simulink model "UR5_SDH_IK"  (R2023b)
settings: Solver=VariableStepAuto  StartTime=0.0  StopTime=10.0  RelTol=1e-3
values from neighbouring files (symbols this model uses):
  R = [1 0 0 ... (first row only)    [Main.m]
  T = transl(P(i,:)) * rpy2tr(0, 0, pi, 'xyz')    [Gluon6L3.m]    (also in Main.m = [     -0.09743  -0.8140    0.5726   -0.1557; UR5_Heart.m = transl(P(i,: )) * rpy2tr(0, pi/4, pi, 'xyz'); drawCircle.m = [R_goal,      P(i,:)')
undefined symbols (not defined in the file or in its folder): smiData, X, Y, Z
libraries: sm_lib x136, fl_lib x25, nesl_utility x14, robotcorelib x2
(part 3 of 3)

== system UR5_SDH_IK/Robot/robot/J6_1_RIGID/x33103_1_RIGID ==
  ReferenceFrame : sm_lib/Frames and Transforms/Reference Frame
  Solid : sm_lib/Body Elements/File Solid  ExtGeomFileName=33103_Default_sldprt.STEP  UnitType=FromFile  ExtGeomFileUnits=m  StepReaderType=HEX  ExportConvexHullGeometry=off  InertiaType=Custom  Mass=smiData.Solid(15).mass  MassUnits=kg  CenterOfMass=smiData.Solid(15).CoM  CenterOfMassUnits=cm  MomentsOfInertia=smiData.Solid(15).MoI  MomentsOfInertiaUnits=kg*cm^2  ProductsOfInertia=smiData.Solid(15).PoI  ProductsOfInertiaUnits=kg*cm^2  BasedOnType=DensityFromFile  Density=1000  DensityUnits=kg/m^3  DoExposeReferenceFrame=on  SerializedFrames=<Frames/>  GraphicType=FromGeometry  MarkerShape=Sphere  MarkerSize=10  GraphicVisPropType=SimpleVisualProperties  GraphicDiffuseColor=smiData.Solid(15).color  GraphicSpecularColor=[0.5 0.5 0.5 1.0]  GraphicAmbientColor=[0.15 0.15 0.15 1.0]  GraphicEmissiveColor=[0.0 0.0 0.0 1.0]  GraphicShininess=75  GraphicOpacity=smiData.Solid(15).opacity
  F : PMIOPort  Side=Left
  connections:
  Solid/RConn1 -- ReferenceFrame/RConn1 -- F/RConn1

== system UR5_SDH_IK/Robot/robot/J6_1_RIGID/x33116_1_RIGID ==
  ReferenceFrame : sm_lib/Frames and Transforms/Reference Frame
  Solid : sm_lib/Body Elements/File Solid  ExtGeomFileName=33116_Default_sldprt.STEP  UnitType=FromFile  ExtGeomFileUnits=m  StepReaderType=HEX  ExportConvexHullGeometry=off  InertiaType=Custom  Mass=smiData.Solid(14).mass  MassUnits=kg  CenterOfMass=smiData.Solid(14).CoM  CenterOfMassUnits=cm  MomentsOfInertia=smiData.Solid(14).MoI  MomentsOfInertiaUnits=kg*cm^2  ProductsOfInertia=smiData.Solid(14).PoI  ProductsOfInertiaUnits=kg*cm^2  BasedOnType=DensityFromFile  Density=1000  DensityUnits=kg/m^3  DoExposeReferenceFrame=on  SerializedFrames=<Frames/>  GraphicType=FromGeometry  MarkerShape=Sphere  MarkerSize=10  GraphicVisPropType=SimpleVisualProperties  GraphicDiffuseColor=smiData.Solid(14).color  GraphicSpecularColor=[0.5 0.5 0.5 1.0]  GraphicAmbientColor=[0.15 0.15 0.15 1.0]  GraphicEmissiveColor=[0.0 0.0 0.0 1.0]  GraphicShininess=75  GraphicOpacity=smiData.Solid(14).opacity
  F : PMIOPort  Side=Left
  connections:
  Solid/RConn1 -- ReferenceFrame/RConn1 -- F/RConn1

== matlab function UR5_SDH_IK/FK/MATLAB Function ==
  data: theta input; T output
function T = zhengyundongxue(theta)
    %已知关节角求变换矩阵
    a=[0,-0.42500,-0.39225,0,0,0];
    d=[0.089159,0,0,0.10915,0.09465,0.08230];
    alpha=[pi/2,0,0,pi/2,-pi/2,0];
 
    
    T01=T_para(theta(1),d(1),a(1),alpha(1));
    T12=T_para(theta(2),d(2),a(2),alpha(2));
    T23=T_para(theta(3),d(3),a(3),alpha(3));
    T34=T_para(theta(4),d(4),a(4),alpha(4));
    T45=T_para(theta(5),d(5),a(5),alpha(5));
    T56=T_para(theta(6),d(6),a(6),alpha(6));
    
    T=T01*T12*T23*T34*T45*T56;
    
end
 
function T = T_para(theta,d,a,alpha)
    T=[ccc(theta),-sss(theta)*ccc(alpha),sss(theta)*sss(alpha),a*ccc(theta);
        sss(theta),ccc(theta)*ccc(alpha),-ccc(theta)*sss(alpha),a*sss(theta);
        0,sss(alpha),ccc(alpha),d;
        0,0,0,1];
end
 
function sss=sss(a)
%     sss=sin(a/180*pi);
    sss=sin(a);
end
 
function ccc=ccc(a)
%     ccc=cos(a/180*pi);
     ccc=cos(a);
end

== matlab function UR5_SDH_IK/MATLAB Function ==
  data: p input; T output; R input
function T = BuildT(p, R)
% BuildT  根据固定旋转矩阵 R 和输入位置 p 构建齐次变换矩阵 T
% 输入:
%   p[3x1] - 末端位置向量 [x; y; z]
% 输出:
%   T[4x4] - 齐次变换矩阵

% 固定旋转矩阵 R
% R = [0, 0, 1;
%      0, -1, 0;
%      1, 0, 0];

% 构建齐次矩阵
T = [R, p(:);     % p(:) 确保为列向量
     0 0 0 1];

end

== matlab function UR5_SDH_IK/MATLAB Function1 ==
  data: T input; joint_angles output
function joint_angles = ur5_inverse_kinematics(T)
%#codegen
%UR5_INVERSE_KINEMATICS UR5机械臂逆运动学解析解（Simulink MATLAB Function兼容）
%
%   输入:  
%       T           - 4x4 齐次变换矩阵，表示末端执行器位姿
%
%   输出:
%       joint_angles - 8x6 矩阵，每行为一组可能的关节角解 [θ1,θ2,θ3,θ4,θ5,θ6] (rad)
%
%   说明:
%       基于UR5标准DH参数:  alpha = [pi/2, 0, 0, pi/2, -pi/2, 0]
%       共有8组解，对应不同的机械臂配置（肩部左/右、肘部上/下、腕部翻转）

    %% ================== UR5 DH参数定义 ==================
    % 连杆长度 (单位: m)
    LINK_A2 = -0.42500;     % 连杆2长度 (上臂)
    LINK_A3 = -0.39225;     % 连杆3长度 (前臂)
    
    % 连杆偏移 (单位: m)
    OFFSET_D1 = 0.089159;   % 基座到关节1的偏移
    OFFSET_D4 = 0.10915;    % 关节3到关节4的偏移
    OFFSET_D5 = 0.09465;    % 关节4到关节5的偏移
    OFFSET_D6 = 0.08230;    % 关节5到末端的偏移

    %% ================== 提取变换矩阵元素 ==================
    % 旋转矩阵 R = [n, o, a]
    % n: 法向量(normal), o: 方向向量(orientation), a: 接近向量(approach)
    nx = T(1,1);  ny = T(2,1);  nz = T(3,1);    % 法向量
    ox = T(1,2);  oy = T(2,2);  oz = T(3,2);    % 方向向量
    ax = T(1,3);  ay = T(2,3);  az = T(3,3);    % 接近向量
    
    % 位置向量 p
    px = T(1,4);  py = T(2,4);  pz = T(3,4);

    %% ================== 初始化所有变量 ==================
    % Simulink代码生成要求：所有数组必须先完整初始化
    joint_angles = zeros(8, 6);
    theta1_sol = zeros(1, 2);
    theta5_sol = zeros(2, 2);
    theta6_sol = zeros(2, 2);
    P14_x = zeros(2, 2);
    P14_z = zeros(2, 2);
    cos_theta3 = zeros(2, 2);
    theta3_sol_pos = zeros(2, 2);
    theta3_sol_neg = zeros(2, 2);
    theta2_sol = zeros(2, 2, 2);

    %% ================== 求解关节角1 (θ1) ==================
    % 计算腕心位置在XY平面的投影
    wrist_center_y = OFFSET_D6 * ay - py;
    wrist_center_x = OFFSET_D6 * ax - px;
    
    % 计算辅助角度和距离
    psi = atan2(wrist_center_y, wrist_center_x);
    
    % 防止数值误差导致负数开方
    dist_squared = wrist_center_x^2 + wrist_center_y^2 - OFFSET_D4^2;
    if dist_squared < 0
        dist_squared = 0;
    end
    radial_dist = sqrt(dist_squared);
    
    % θ1的两个解 (左肩/右肩配置)
    theta1_sol(1) = psi - atan2(OFFSET_D4,  radial_dist);
    theta1_sol(2) = psi - atan2(OFFSET_D4, -radial_dist);

    %% ================== 求解关节角5 (θ5) ==================
    % 对每个θ1计算θ5
    cos_theta5_1 = ax * sin(theta1_sol(1)) - ay * cos(theta1_sol(1));
    cos_theta5_2 = ax * sin(theta1_sol(2)) - ay * cos(theta1_sol(2));
    
    % 限制cos值在[-1, 1]范围内
    if cos_theta5_1 > 1
        cos_theta5_1 = 1;
    elseif cos_theta5_1 < -1
        cos_theta5_1 = -1;
    end
    
    if cos_theta5_2 > 1
        cos_theta5_2 = 1;
    elseif cos_theta5_2 < -1
        cos_theta5_2 = -1;
    end
    
    % θ5的四个解 (腕部正/反配置)
    % theta5_sol(i,j): i=1,2对应θ1的两个解, j=1,2对应θ5的正负解
    theta5_sol(1,1) =  acos(cos_theta5_1);    % θ1解1, θ5正
    theta5_sol(1,2) = -acos(cos_theta5_1);    % θ1解1, θ5负
    theta5_sol(2,1) =  acos(cos_theta5_2);    % θ1解2, θ5正
    theta5_sol(2,2) = -acos(cos_theta5_2);    % θ1解2, θ5负

    %% ================== 求解关节角6 (θ6) ==================
    % 计算中间变量
    sin_theta6_base1 = nx * sin(theta1_sol(1)) - ny * cos(theta1_sol(1));
    cos_theta6_base1 = ox * sin(theta1_sol(1)) - oy * cos(theta1_sol(1));
    sin_theta6_base2 = nx * sin(theta1_sol(2)) - ny * cos(theta1_sol(2));
    cos_theta6_base2 = ox * sin(theta1_sol(2)) - oy * cos(theta1_sol(2));
    
    % θ6的四个解
    theta6_sol(1,1) = atan2(sin_theta6_base1, cos_theta6_base1) - atan2(sin(theta5_sol(1,1)), 0);
    theta6_sol(1,2) = atan2(sin_theta6_base1, cos_theta6_base1) - atan2(sin(theta5_sol(1,2)), 0);
    theta6_sol(2,1) = atan2(sin_theta6_base2, cos_theta6_base2) - atan2(sin(theta5_sol(2,1)), 0);
    theta6_sol(2,2) = atan2(sin_theta6_base2, cos_theta6_base2) - atan2(sin(theta5_sol(2,2)), 0);

    %% ================== 求解关节角3 (θ3) ==================
    % 计算腕部在关节1坐标系下的位置投影
    for i = 1:2      % 遍历θ1的两个解
        for j = 1:2  % 遍历θ5/θ6的两个解
            c1 = cos(theta1_sol(i));
            s1 = sin(theta1_sol(i));
            c6 = cos(theta6_sol(i,j));
            s6 = sin(theta6_sol(i,j));
            
            % 腕部位置x分量
            P14_x(i,j) = OFFSET_D5 * (s6 * (nx*c1 + ny*s1) + c6 * (ox*c1 + oy*s1)) ... 
                       - OFFSET_D6 * (ax*c1 + ay*s1) + px*c1 + py*s1;
            
            % 腕部位置z分量
            P14_z(i,j) = pz - OFFSET_D1 - az*OFFSET_D6 + OFFSET_D5 * (oz*c6 + nz*s6);
        end
    end
    
    % 使用余弦定理求解θ3
    for i = 1:2
        for j = 1:2
            numerator = P14_x(i,j)^2 + P14_z(i,j)^2 - LINK_A2^2 - LINK_A3^2;
            denominator = 2 * LINK_A2 * LINK_A3;
            cos_theta3(i,j) = numerator / denominator;
            
            % 限制cos值范围
            if cos_theta3(i,j) > 1
                cos_theta3(i,j) = 1;
            elseif cos_theta3(i,j) < -1
                cos_theta3(i,j) = -1;
            end
            
            theta3_sol_pos(i,j) =  acos(cos_theta3(i,j));
            theta3_sol_neg(i,j) = -acos(cos_theta3(i,j));
        end
    end

    %% ================== 求解关节角2 (θ2) ==================
    for i = 1:2
        for j = 1:2
            % θ3为正解时的θ2
            theta2_sol(i,j,1) = calc_theta2_inline(P14_x(i,j), P14_z(i,j), ...
                                                   theta3_sol_pos(i,j), LINK_A2, LINK_A3);
            % θ3为负解时的θ2
            theta2_sol(i,j,2) = calc_theta2_inline(P14_x(i,j), P14_z(i,j), ...
                                                   theta3_sol_neg(i,j), LINK_A2, LINK_A3);
        end
    end

    %% ================== 组装8组解 ==================
    solution_idx = 1;
    for i = 1:2          % θ1索引
        for j = 1:2      % θ5索引
            for k = 1:2  % θ3正负索引
                % 选择对应的θ3
                if k == 1
                    theta3_val = theta3_sol_pos(i,j);
                else
                    theta3_val = theta3_sol_neg(i,j);
                end
                
                % 赋值 θ1, θ2, θ3
                joint_angles(solution_idx, 1) = theta1_sol(i);
                joint_angles(solution_idx, 2) = theta2_sol(i,j,k);
                joint_angles(solution_idx, 3) = theta3_val;
                
                % 赋值 θ5, θ6
                joint_angles(solution_idx, 5) = theta5_sol(i,j);
                joint_angles(solution_idx, 6) = theta6_sol(i,j);
                
                solution_idx = solution_idx + 1;
            end
        end
    end

    %% ================== 求解关节角4 (θ4) ==================
    for sol = 1:8
        t1 = joint_angles(sol, 1);
        t2 = joint_angles(sol, 2);
        t3 = joint_angles(sol, 3);
        t6 = joint_angles(sol, 6);
        
        c1 = cos(t1);
        s1 = sin(t1);
        c6 = cos(t6);
        s6 = sin(t6);
        
        % 计算θ4的sin和cos分量
        sin_theta234 = -s6 * (nx*c1 + ny*s1) - c6 * (ox*c1 + oy*s1);
        cos_theta234 = oz*c6 + nz*s6;
        
        theta234 = atan2(sin_theta234, cos_theta234);
        joint_angles(sol, 4) = theta234 - t2 - t3;
    end

    %% ================== 角度归一化 ==================
    for sol = 1:8
        for jnt = 1:6
            ang = joint_angles(sol, jnt);
            while ang > pi
                ang = ang - 2*pi;
            end
            while ang < -pi
                ang = ang + 2*pi;
            end
            joint_angles(sol, jnt) = ang;
        end
    end

end

%% ================== 内联函数:  计算θ2 ==================
function theta2 = calc_theta2_inline(P14_x, P14_z, theta3, A2, A3)
%CALC_THETA2_INLINE 根据几何关系计算关节角2

    c3 = cos(theta3);
    s3 = sin(theta3);
    
    % 分母
    denom = A2^2 + A3^2 + 2*A2*A3*c3;
    
    % 防止除零
    if abs(denom) < 1e-10
        denom = 1e-10;
    end
    
    % 计算sin(θ2)和cos(θ2)
    sin_theta2 = ((A3*c3 + A2) * P14_z - A3*s3 * P14_x) / denom;
    
    % 防止除零
    denom2 = A3*c3 + A2;
    if abs(denom2) < 1e-10
        denom2 = 1e-10;
    end
    cos_theta2 = (P14_x + A3*s3 * sin_theta2) / denom2;
    
    theta2 = atan2(sin_theta2, cos_theta2);
end

== matlab function UR5_SDH_IK/MATLAB Function2 ==
  data: all_solutions input; optimal_joint output; current_joint input
function optimal_joint = ur5_select_optimal_simple(all_solutions, current_joint)
%#codegen
%UR5_SELECT_OPTIMAL_SIMPLE 从8组逆解中选择最优解（简化版）
%
%   输入:
%       all_solutions - 8x6 矩阵，8组可能的关节角解 (rad)
%       current_joint - 1x6 向量，当前关节角度 (rad)
%
%   输出:
%       optimal_joint - 1x6 向量，最优的关节角解 (rad)
%
%   选择准则:  选择与当前关节角度变化最小的有效解

    %% ================== 初始化 ==================
    NUM_SOLUTIONS = 8;
    NUM_JOINTS = 6;
    
    optimal_joint = zeros(1, NUM_JOINTS);
    min_distance = 1e10;
    best_idx = 0;

    %% ================== 遍历所有解 ==================
    for sol_idx = 1:NUM_SOLUTIONS
        
        % 检查是否为有效解（无NaN/Inf）
        is_valid = true;
        for j = 1:NUM_JOINTS
            if isnan(all_solutions(sol_idx, j)) || isinf(all_solutions(sol_idx, j))
                is_valid = false;
            end
        end
        
        if ~is_valid
            continue;
        end
        
        % 计算与当前关节角度的距离
        distance = 0;
        for j = 1:NUM_JOINTS
            % 角度差归一化
            diff = all_solutions(sol_idx, j) - current_joint(j);
            
            while diff > pi
                diff = diff - 2*pi;
            end
            while diff < -pi
                diff = diff + 2*pi;
            end
            
            distance = distance + diff^2;
        end
        distance = sqrt(distance);
        
        % 更新最优解
        if distance < min_distance
            min_distance = distance;
            best_idx = sol_idx;
        end
    end

    %% ================== 输出结果 ==================
    if best_idx > 0
        for j = 1:NUM_JOINTS
            ang = all_solutions(best_idx, j);
            while ang > pi
                ang = ang - 2*pi;
            end
            while ang < -pi
                ang = ang + 2*pi;
            end
            optimal_joint(j) = ang;
        end
    else
        % 无有效解，返回当前角度
        for j = 1:NUM_JOINTS
            optimal_joint(j) = current_joint(j);
        end
    end

end

== matlab function UR5_SDH_IK/MATLAB Function3 ==
  data: theta input; T output
function T = zhengyundongxue(theta)
    %已知关节角求变换矩阵
    a=[0,-0.42500,-0.39225,0,0,0];
    d=[0.089159,0,0,0.10915,0.09465,0.08230];
    alpha=[pi/2,0,0,pi/2,-pi/2,0];
 
    
    T01=T_para(theta(1),d(1),a(1),alpha(1));
    T12=T_para(theta(2),d(2),a(2),alpha(2));
    T23=T_para(theta(3),d(3),a(3),alpha(3));
    T34=T_para(theta(4),d(4),a(4),alpha(4));
    T45=T_para(theta(5),d(5),a(5),alpha(5));
    T56=T_para(theta(6),d(6),a(6),alpha(6));
    
    T=T01*T12*T23*T34*T45*T56;
    
end
 
function T = T_para(theta,d,a,alpha)
    T=[ccc(theta),-sss(theta)*ccc(alpha),sss(theta)*sss(alpha),a*ccc(theta);
        sss(theta),ccc(theta)*ccc(alpha),-ccc(theta)*sss(alpha),a*sss(theta);
        0,sss(alpha),ccc(alpha),d;
        0,0,0,1];
end
 
function sss=sss(a)
%     sss=sin(a/180*pi);
    sss=sin(a);
end
 
function ccc=ccc(a)
%     ccc=cos(a/180*pi);
     ccc=cos(a);
end
